simulink model "PID_Test"  (R2015b)
settings: Solver=VariableStepAuto  StartTime=0.0  StopTime=10  FixedStep=0.1  RelTol=1e-3
InitFcn:
  | fs = 50 % 50Hz sampleling frequency
  | g = 9.81 % gravity
undefined symbols (not defined in the file or in its folder): D1, D2, I1
libraries: simulink x3
settings Model: Creator=freddiesherratt  LastModifiedBy=fs349

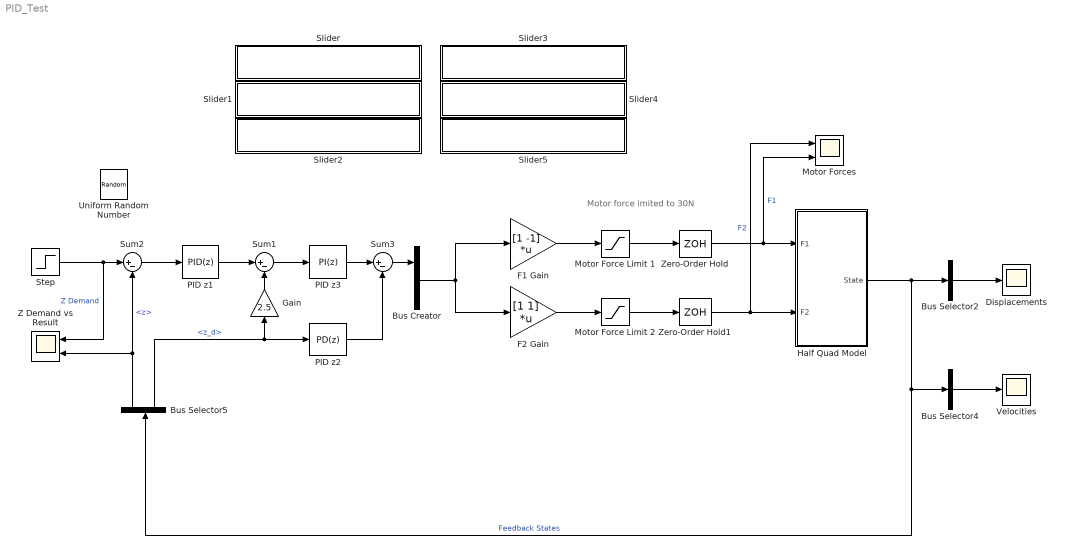
== system PID_Test ==
  note: Motor force
      | imited to 30N
  Bus Creator : BusCreator  Inputs=2
  Bus Selector2 : BusSelector  OutputSignals=z,x,beta  OutputAsBus=on
  Bus Selector4 : BusSelector  OutputSignals=z_d,x_dd,beta_d  OutputAsBus=on
  Bus Selector5 : BusSelector  OutputSignals=z,z_d
  Displacements : Scope
  F1 Gain : Gain  Gain=[1 -1]  Multiplication=Matrix(K*u)
  F2 Gain : Gain  Gain=[1 1]  Multiplication=Matrix(K*u)
  Gain : Gain  Gain=2.5
  Half Quad Model : Subsystem  mask{m=0.25, I=0.1, a=1, g=g}
      mask prompts: m "m, Mass (Kg)"; I "I, Intertia (Kg m^2)"; a "a, moment arm lenght (m)"; g "g, Gravity (ms^2)"
  Motor Force Limit 1 : Saturate  UpperLimit=30  LowerLimit=0
  Motor Force Limit 2 : Saturate  UpperLimit=30  LowerLimit=0
  Motor Forces : Scope  NumInputPorts=2
  PID z1 : simulink/Continuous/PID Controller  Controller=PID  TimeDomain=Discrete-time  SampleTime=1/fs  IntegratorMethod=Forward Euler  FilterMethod=Forward Euler  Form=Parallel  UseFilter=off  ControllerParametersSource=internal  P=11.4  I=0  D=D1  N=32518.3816607502  InitialConditionSource=internal  InitialConditionForIntegrator=0  InitialConditionForFilter=0  ExternalReset=none  LimitOutput=off  UpperSaturationLimit=inf  LowerSaturationLimit=-inf  LinearizeAsGain=on  AntiWindupMode=none  Kb=1  TrackingMode=off  Kt=1  PParamMin=[]  PParamMax=[]  IParamMin=[]  IParamMax=[]  DParamMin=[]  DParamMax=[]  NParamMin=[]  NParamMax=[]  KbParamMin=[]  KbParamMax=[]  KtParamMin=[]  KtParamMax=[]  POutMin=[]  POutMax=[]  IOutMin=[]  IOutMax=[]  DOutMin=[]  DOutMax=[]  NOutMin=[]  NOutMax=[]  KbOutMin=[]  KbOutMax=[]  KtOutMin=[]  KtOutMax=[]  IntegratorOutMin=[]  IntegratorOutMax=[]  FilterOutMin=[]  FilterOutMax=[]  SumOutMin=[]  SumOutMax=[]  SumI1OutMin=[]  SumI1OutMax=[]  SumI2OutMin=[]  SumI2OutMax=[]  SumI3OutMin=[]  SumI3OutMax=[]  SumDOutMin=[]  SumDOutMax=[]  SaturationOutMin=[]  SaturationOutMax=[]  IntegratorContinuousStateAttributes=''  IntegratorStateMustResolveToSignalObject=off  IntegratorRTWStateStorageClass=Auto  FilterContinuousStateAttributes=''  FilterStateMustResolveToSignalObject=off  FilterRTWStateStorageClass=Auto  DifferentiatorICPrevScaledInput=0  DifferentiatorOutMin=[]  DifferentiatorOutMax=[]
  PID z2 : simulink/Continuous/PID Controller  Controller=PD  TimeDomain=Discrete-time  SampleTime=1/fs  IntegratorMethod=Forward Euler  FilterMethod=Forward Euler  Form=Parallel  UseFilter=off  ControllerParametersSource=internal  P=0  I=I1  D=0.2  N=32518.3816607502  InitialConditionSource=internal  InitialConditionForIntegrator=0  InitialConditionForFilter=0  ExternalReset=none  LimitOutput=off  UpperSaturationLimit=inf  LowerSaturationLimit=-inf  LinearizeAsGain=on  AntiWindupMode=none  Kb=1  TrackingMode=off  Kt=1  PParamMin=[]  PParamMax=[]  IParamMin=[]  IParamMax=[]  DParamMin=[]  DParamMax=[]  NParamMin=[]  NParamMax=[]  KbParamMin=[]  KbParamMax=[]  KtParamMin=[]  KtParamMax=[]  POutMin=[]  POutMax=[]  IOutMin=[]  IOutMax=[]  DOutMin=[]  DOutMax=[]  NOutMin=[]  NOutMax=[]  KbOutMin=[]  KbOutMax=[]  KtOutMin=[]  KtOutMax=[]  IntegratorOutMin=[]  IntegratorOutMax=[]  FilterOutMin=[]  FilterOutMax=[]  SumOutMin=[]  SumOutMax=[]  SumI1OutMin=[]  SumI1OutMax=[]  SumI2OutMin=[]  SumI2OutMax=[]  SumI3OutMin=[]  SumI3OutMax=[]  SumDOutMin=[]  SumDOutMax=[]  SaturationOutMin=[]  SaturationOutMax=[]  IntegratorContinuousStateAttributes=''  IntegratorStateMustResolveToSignalObject=off  IntegratorRTWStateStorageClass=Auto  FilterContinuousStateAttributes=''  FilterStateMustResolveToSignalObject=off  FilterRTWStateStorageClass=Auto  DifferentiatorICPrevScaledInput=0  DifferentiatorOutMin=[]  DifferentiatorOutMax=[]
  PID z3 : simulink/Continuous/PID Controller  Controller=PI  TimeDomain=Discrete-time  SampleTime=1/fs  IntegratorMethod=Forward Euler  FilterMethod=Forward Euler  Form=Parallel  UseFilter=off  ControllerParametersSource=internal  P=2  I=0  D=D2  N=32518.3816607502  InitialConditionSource=internal  InitialConditionForIntegrator=0  InitialConditionForFilter=0  ExternalReset=none  LimitOutput=off  UpperSaturationLimit=inf  LowerSaturationLimit=-inf  LinearizeAsGain=on  AntiWindupMode=none  Kb=1  TrackingMode=off  Kt=1  PParamMin=[]  PParamMax=[]  IParamMin=[]  IParamMax=[]  DParamMin=[]  DParamMax=[]  NParamMin=[]  NParamMax=[]  KbParamMin=[]  KbParamMax=[]  KtParamMin=[]  KtParamMax=[]  POutMin=[]  POutMax=[]  IOutMin=[]  IOutMax=[]  DOutMin=[]  DOutMax=[]  NOutMin=[]  NOutMax=[]  KbOutMin=[]  KbOutMax=[]  KtOutMin=[]  KtOutMax=[]  IntegratorOutMin=[]  IntegratorOutMax=[]  FilterOutMin=[]  FilterOutMax=[]  SumOutMin=[]  SumOutMax=[]  SumI1OutMin=[]  SumI1OutMax=[]  SumI2OutMin=[]  SumI2OutMax=[]  SumI3OutMin=[]  SumI3OutMax=[]  SumDOutMin=[]  SumDOutMax=[]  SaturationOutMin=[]  SaturationOutMax=[]  IntegratorContinuousStateAttributes=''  IntegratorStateMustResolveToSignalObject=off  IntegratorRTWStateStorageClass=Auto  FilterContinuousStateAttributes=''  FilterStateMustResolveToSignalObject=off  FilterRTWStateStorageClass=Auto  DifferentiatorICPrevScaledInput=0  DifferentiatorOutMin=[]  DifferentiatorOutMax=[]
  Slider : Subsystem  DialogController=hmiCreateDDGDialog  IsWebBlock=on  mask(MWDashboardBlock){webBlockId=fd489732-8b6d-419f-b239-95cad41e5fc3, webBlockType=slider, ShowInLibBrowser=on, ShowInitialText=on, HMISrcModelName=PID_Test}
      mask prompts: webBlockId "WebBlock Id"; webBlockType "WebBlock Type"; HMISrcModelName "Source Model"
      mask Help: helpview([docroot '/mapfiles/simulink.map'], 'hmi_slider')
      mask Display:
      | if strcmp(get_param(bdroot(gcb),'BlockDiagramType'), 'library')
      |     image([(matlabroot) '/toolbox/simulink/hmi/icons/Slider.png']);
      | end
  Slider1 : Subsystem  DialogController=hmiCreateDDGDialog  IsWebBlock=on  mask(MWDashboardBlock){webBlockId=a2dd80f1-a299-4775-96c0-e436f38ab54b, webBlockType=slider, ShowInLibBrowser=on, ShowInitialText=on, HMISrcModelName=PID_Test}
      mask prompts: webBlockId "WebBlock Id"; webBlockType "WebBlock Type"; HMISrcModelName "Source Model"
      mask Help: helpview([docroot '/mapfiles/simulink.map'], 'hmi_slider')
      mask Display:
      | if strcmp(get_param(bdroot(gcb),'BlockDiagramType'), 'library')
      |     image([(matlabroot) '/toolbox/simulink/hmi/icons/Slider.png']);
      | end
  Slider2 : Subsystem  DialogController=hmiCreateDDGDialog  IsWebBlock=on  mask(MWDashboardBlock){webBlockId=b22de405-6f97-459f-a33c-a68948852966, webBlockType=slider, ShowInLibBrowser=on, ShowInitialText=on, HMISrcModelName=PID_Test}
      mask prompts: webBlockId "WebBlock Id"; webBlockType "WebBlock Type"; HMISrcModelName "Source Model"
      mask Help: helpview([docroot '/mapfiles/simulink.map'], 'hmi_slider')
      mask Display:
      | if strcmp(get_param(bdroot(gcb),'BlockDiagramType'), 'library')
      |     image([(matlabroot) '/toolbox/simulink/hmi/icons/Slider.png']);
      | end
  Slider3 : Subsystem  DialogController=hmiCreateDDGDialog  IsWebBlock=on  mask(MWDashboardBlock){webBlockId=34e38c82-e8d5-44d4-b0cb-519f02bd1da9, webBlockType=slider, ShowInLibBrowser=on, ShowInitialText=on, HMISrcModelName=PID_Test}
      mask prompts: webBlockId "WebBlock Id"; webBlockType "WebBlock Type"; HMISrcModelName "Source Model"
      mask Help: helpview([docroot '/mapfiles/simulink.map'], 'hmi_slider')
      mask Display:
      | if strcmp(get_param(bdroot(gcb),'BlockDiagramType'), 'library')
      |     image([(matlabroot) '/toolbox/simulink/hmi/icons/Slider.png']);
      | end
  Slider4 : Subsystem  DialogController=hmiCreateDDGDialog  IsWebBlock=on  mask(MWDashboardBlock){webBlockId=4711e98c-76f4-4d7a-a591-9a326a98a612, webBlockType=slider, ShowInLibBrowser=on, ShowInitialText=on, HMISrcModelName=PID_Test}
      mask prompts: webBlockId "WebBlock Id"; webBlockType "WebBlock Type"; HMISrcModelName "Source Model"
      mask Help: helpview([docroot '/mapfiles/simulink.map'], 'hmi_slider')
      mask Display:
      | if strcmp(get_param(bdroot(gcb),'BlockDiagramType'), 'library')
      |     image([(matlabroot) '/toolbox/simulink/hmi/icons/Slider.png']);
      | end
  Slider5 : Subsystem  DialogController=hmiCreateDDGDialog  IsWebBlock=on  mask(MWDashboardBlock){webBlockId=bb9a2908-5384-43ba-984c-02658a67681d, webBlockType=slider, ShowInLibBrowser=on, ShowInitialText=on, HMISrcModelName=PID_Test}
      mask prompts: webBlockId "WebBlock Id"; webBlockType "WebBlock Type"; HMISrcModelName "Source Model"
      mask Help: helpview([docroot '/mapfiles/simulink.map'], 'hmi_slider')
      mask Display:
      | if strcmp(get_param(bdroot(gcb),'BlockDiagramType'), 'library')
      |     image([(matlabroot) '/toolbox/simulink/hmi/icons/Slider.png']);
      | end
  Step : Step  SampleTime=0
  Sum1 : Sum  Inputs=|+-
  Sum2 : Sum  Inputs=|+-
  Sum3 : Sum  Inputs=|+-
  Uniform Random Number : UniformRandomNumber  Minimum=0  SampleTime=0.8
  Velocities : Scope
  Z Demand vs Result : Scope  NumInputPorts=2
  Zero-Order Hold : ZeroOrderHold  SampleTime=1/fs
  Zero-Order Hold1 : ZeroOrderHold  SampleTime=1/fs
  wires:
  Step/1 -> Sum2/1, Z Demand vs Result/1  "Z Demand"
  F2 Gain/1 -> Motor Force Limit 2/1
  Motor Force Limit 2/1 -> Zero-Order Hold1/1
  Motor Force Limit 1/1 -> Zero-Order Hold/1
  F1 Gain/1 -> Motor Force Limit 1/1
  Bus Creator/1 -> F2 Gain/1, F1 Gain/1
  Bus Selector2/1 -> Displacements/1
  Zero-Order Hold/1 -> Motor Forces/2, Half Quad Model/1(F1)  "F1"
  Zero-Order Hold1/1 -> Motor Forces/1, Half Quad Model/2(F2)  "F2"
  Half Quad Model/1(State) -> Bus Selector2/1, Bus Selector4/1, Bus Selector5/1  "Feedback States"
  Bus Selector5/1 -> Z Demand vs Result/2, Sum2/2  "<z>"
  Bus Selector4/1 -> Velocities/1
  Sum1/1 -> PID z3/1
  Sum2/1 -> PID z1/1
  PID z1/1 -> Sum1/1
  Bus Selector5/2 -> PID z2/1, Gain/1  "<z_d>"
  PID z2/1 -> Sum3/2
  Gain/1 -> Sum1/2
  Sum3/1 -> Bus Creator/1
  PID z3/1 -> Sum3/1

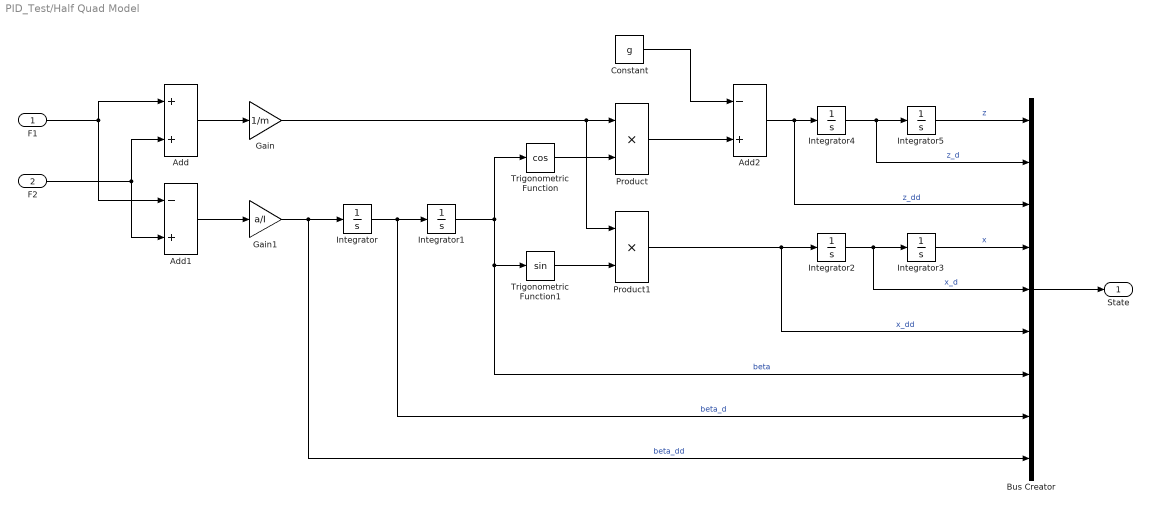
== system PID_Test/Half Quad Model ==
  F1 : Inport
  F2 : Inport  Port=2
  Add : Sum
  Add1 : Sum  Inputs=-+
  Add2 : Sum  Inputs=-+
  Bus Creator : BusCreator  Inputs=9
  Constant : Constant  Value=g
  Gain : Gain  Gain=1/m
  Gain1 : Gain  Gain=a/I
  Integrator{,1..5} (6 alike) : Integrator
  Product : Product
  Product1 : Product
  Trigonometric Function : Trigonometry  Operator=cos
  Trigonometric Function1 : Trigonometry
  State : Outport
  wires:
  Integrator1/1 -> Trigonometric Function/1, Trigonometric Function1/1, Bus Creator/7  "beta"
  F2/1 -> Add/2, Add1/2
  Add/1 -> Gain/1
  Gain/1 -> Product/1, Product1/1
  Integrator/1 -> Bus Creator/8, Integrator1/1  "beta_d"
  Product/1 -> Add2/2
  Integrator4/1 -> Integrator5/1, Bus Creator/2  "z_d"
  Trigonometric Function/1 -> Product/2
  Gain1/1 -> Bus Creator/9, Integrator/1  "beta_dd"
  Trigonometric Function1/1 -> Product1/2
  F1/1 -> Add1/1, Add/1
  Constant/1 -> Add2/1
  Product1/1 -> Bus Creator/6, Integrator2/1  "x_dd"
  Integrator5/1 -> Bus Creator/1  "z"
  Add2/1 -> Integrator4/1, Bus Creator/3  "z_dd"
  Bus Creator/1 -> State/1
  Integrator3/1 -> Bus Creator/4  "x"
  Integrator2/1 -> Integrator3/1, Bus Creator/5  "x_d"
  Add1/1 -> Gain1/1

== system PID_Test/Slider ==

== system PID_Test/Slider1 ==

== system PID_Test/Slider2 ==

== system PID_Test/Slider3 ==

== system PID_Test/Slider4 ==

== system PID_Test/Slider5 ==
